simulink model "monitor"  (R2022a)
settings: Solver=FixedStepDiscrete  StartTime=0.0  StopTime=simTime  RelTol=1e-3
libraries: dspsrcs4 x16
settings Model: DataTypeOverride=Off  Creator=alpha  LastModifiedBy=alpha
settings SolverCC: AlgebraicLoopSolver=TrustRegion
settings DataIOCC: LimitDataPoints=on  SaveOutput=off  SaveTime=off
settings OptimizationCC: BlockReduction=off  ConditionallyExecuteInputs=off  DefaultParameterBehavior=Inlined  LifeSpan=inf
settings DebuggingCC: AlgebraicLoopMsg=error  SingleTaskRateTransMsg=error  UnconnectedInputMsg=warning  UnconnectedOutputMsg=warning  UnconnectedLineMsg=warning  AllowSymbolicDim=off  StrictBusMsg=ErrorOnBusTreatedAsVector  SFUnexpectedBacktrackingDiag=warning  SFNoUnconditionalDefaultTransitionDiag=warning  SFExecutionAtInitializationDiag=none  SFMachineParentedDataDiag=warning  ArithmeticOperatorsInVariantConditions=warning
settings HardwareCC: ProdBitPerPointer=32  ProdBitPerSizeT=32  ProdBitPerPtrDiffT=32  ProdLargestAtomicFloat=None  ProdIntDivRoundTo=Undefined  ProdEndianess=Unspecified  ProdWordSize=32  ProdHWDeviceType=ASIC/FPGA->ASIC/FPGA  ProdEqTarget=off
settings SFSimCC: SimUseLocalCustomCode=off  CustomCodeUndefinedFunction=UseInterfaceOnly
settings RTWCC: RTWUseLocalCustomCode=off
settings CodeAppCC: StateflowObjectComments=on
settings GRTTargetCC: TargetLangStandard=C89/C90 (ANSI)
settings ConfigComp: CovScope=ReferencedModels  CovMetricSettings=dw  CovSaveCumulativeToWorkspaceVar=on  CovSaveSingleToWorkspaceVar=on  CovExternalEMLEnable=off  CovSFcnEnable=off

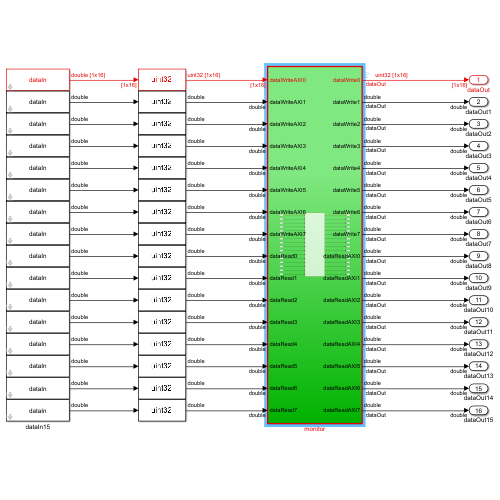
[thumbnail: Simulink's stored preview of the top-level diagram]
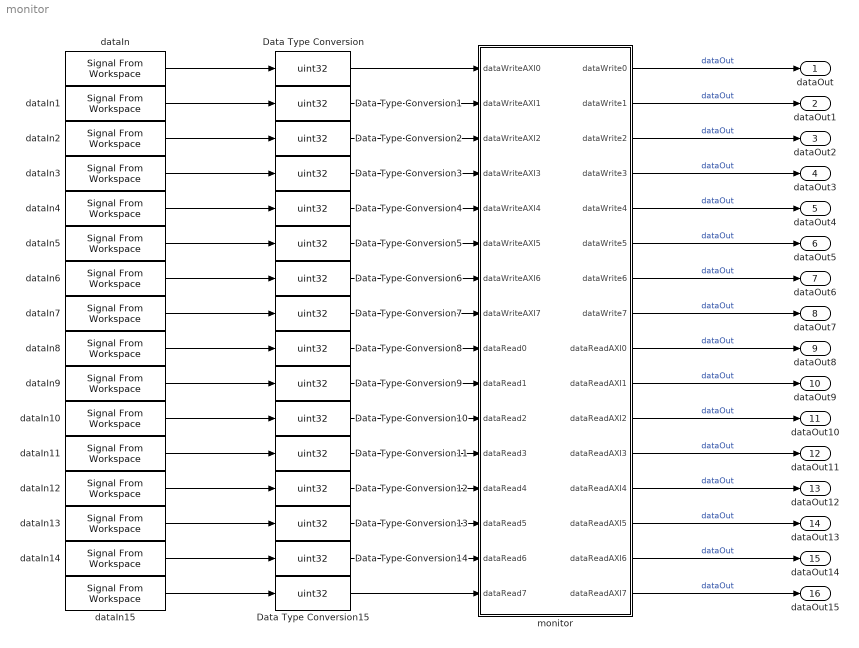
== system monitor ==
  Data Type Conversion{,1..15} (16 alike) : DataTypeConversion  OutDataTypeStr=uint32  SaturateOnIntegerOverflow=off  RndMeth=Floor
  dataIn{,1..15} (16 alike) : dspsrcs4/Signal From Workspace  X=dataIn  Ts=1  nsamps=1  OutputAfterFinalValue=Setting to zero  ignoreOrWarnInputAndFrameLengths=off  OutputFrames=off
  monitor : Subsystem  TreatAsAtomicUnit=on
  dataOut : Outport
  dataOut1 : Outport  Port=2
  dataOut2 : Outport  Port=3
  dataOut3 : Outport  Port=4
  dataOut4 : Outport  Port=5
  dataOut5 : Outport  Port=6
  dataOut6 : Outport  Port=7
  dataOut7 : Outport  Port=8
  dataOut8 : Outport  Port=9
  dataOut9 : Outport  Port=10
  dataOut10 : Outport  Port=11
  dataOut11 : Outport  Port=12
  dataOut12 : Outport  Port=13
  dataOut13 : Outport  Port=14
  dataOut14 : Outport  Port=15
  dataOut15 : Outport  Port=16
  wires:
  dataIn/1 -> Data Type Conversion/1
  Data Type Conversion/1 -> monitor/1(dataWriteAXI0)
  monitor/1(dataWrite0) -> dataOut/1  "dataOut"
  monitor/2(dataWrite1) -> dataOut1/1  "dataOut"
  monitor/3(dataWrite2) -> dataOut2/1  "dataOut"
  monitor/4(dataWrite3) -> dataOut3/1  "dataOut"
  monitor/8(dataWrite7) -> dataOut7/1  "dataOut"
  monitor/6(dataWrite5) -> dataOut5/1  "dataOut"
  monitor/5(dataWrite4) -> dataOut4/1  "dataOut"
  monitor/7(dataWrite6) -> dataOut6/1  "dataOut"
  monitor/14(dataReadAXI5) -> dataOut13/1  "dataOut"
  monitor/15(dataReadAXI6) -> dataOut14/1  "dataOut"
  monitor/12(dataReadAXI3) -> dataOut11/1  "dataOut"
  monitor/10(dataReadAXI1) -> dataOut9/1  "dataOut"
  monitor/16(dataReadAXI7) -> dataOut15/1  "dataOut"
  monitor/13(dataReadAXI4) -> dataOut12/1  "dataOut"
  monitor/9(dataReadAXI0) -> dataOut8/1  "dataOut"
  monitor/11(dataReadAXI2) -> dataOut10/1  "dataOut"
  dataIn1/1 -> Data Type Conversion1/1
  Data Type Conversion1/1 -> monitor/2(dataWriteAXI1)
  Data Type Conversion3/1 -> monitor/4(dataWriteAXI3)
  dataIn2/1 -> Data Type Conversion2/1
  Data Type Conversion2/1 -> monitor/3(dataWriteAXI2)
  dataIn3/1 -> Data Type Conversion3/1
  Data Type Conversion5/1 -> monitor/6(dataWriteAXI5)
  dataIn6/1 -> Data Type Conversion6/1
  Data Type Conversion7/1 -> monitor/8(dataWriteAXI7)
  Data Type Conversion6/1 -> monitor/7(dataWriteAXI6)
  dataIn4/1 -> Data Type Conversion4/1
  dataIn5/1 -> Data Type Conversion5/1
  dataIn7/1 -> Data Type Conversion7/1
  Data Type Conversion4/1 -> monitor/5(dataWriteAXI4)
  dataIn15/1 -> Data Type Conversion15/1
  Data Type Conversion9/1 -> monitor/10(dataRead1)
  dataIn13/1 -> Data Type Conversion13/1
  dataIn14/1 -> Data Type Conversion14/1
  Data Type Conversion13/1 -> monitor/14(dataRead5)
  Data Type Conversion12/1 -> monitor/13(dataRead4)
  Data Type Conversion15/1 -> monitor/16(dataRead7)
  Data Type Conversion14/1 -> monitor/15(dataRead6)
  dataIn10/1 -> Data Type Conversion10/1
  Data Type Conversion11/1 -> monitor/12(dataRead3)
  dataIn8/1 -> Data Type Conversion8/1
  Data Type Conversion10/1 -> monitor/11(dataRead2)
  dataIn9/1 -> Data Type Conversion9/1
  dataIn11/1 -> Data Type Conversion11/1
  dataIn12/1 -> Data Type Conversion12/1
  Data Type Conversion8/1 -> monitor/9(dataRead0)

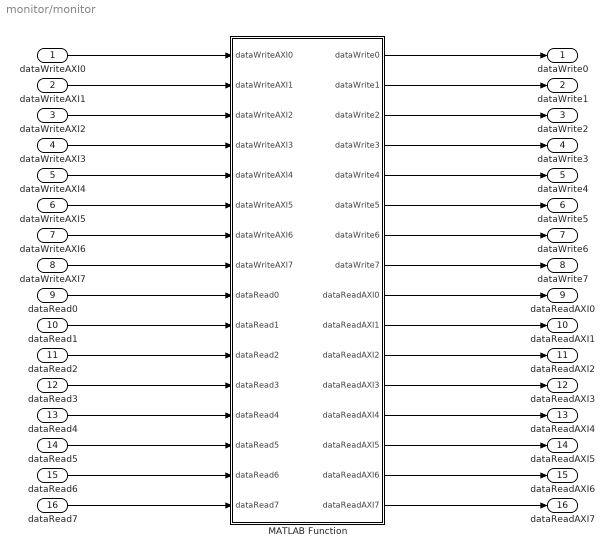
== system monitor/monitor ==
  dataWriteAXI0 : Inport
  dataWriteAXI1 : Inport  Port=2
  dataWriteAXI2 : Inport  Port=3
  dataWriteAXI3 : Inport  Port=4
  dataWriteAXI4 : Inport  Port=5
  dataWriteAXI5 : Inport  Port=6
  dataWriteAXI6 : Inport  Port=7
  dataWriteAXI7 : Inport  Port=8
  dataRead0 : Inport  Port=9
  dataRead1 : Inport  Port=10
  dataRead2 : Inport  Port=11
  dataRead3 : Inport  Port=12
  dataRead4 : Inport  Port=13
  dataRead5 : Inport  Port=14
  dataRead6 : Inport  Port=15
  dataRead7 : Inport  Port=16
  MATLAB Function : MATLAB Function  TreatAsAtomicUnit=on
  dataWrite0 : Outport
  dataWrite1 : Outport  Port=2
  dataWrite2 : Outport  Port=3
  dataWrite3 : Outport  Port=4
  dataWrite4 : Outport  Port=5
  dataWrite5 : Outport  Port=6
  dataWrite6 : Outport  Port=7
  dataWrite7 : Outport  Port=8
  dataReadAXI0 : Outport  Port=9
  dataReadAXI1 : Outport  Port=10
  dataReadAXI2 : Outport  Port=11
  dataReadAXI3 : Outport  Port=12
  dataReadAXI4 : Outport  Port=13
  dataReadAXI5 : Outport  Port=14
  dataReadAXI6 : Outport  Port=15
  dataReadAXI7 : Outport  Port=16
  wires:
  dataWriteAXI0/1 -> MATLAB Function/1(dataWriteAXI0)
  MATLAB Function/1(dataWrite0) -> dataWrite0/1
  dataWriteAXI1/1 -> MATLAB Function/2(dataWriteAXI1)
  dataWriteAXI2/1 -> MATLAB Function/3(dataWriteAXI2)
  dataWriteAXI3/1 -> MATLAB Function/4(dataWriteAXI3)
  dataWriteAXI4/1 -> MATLAB Function/5(dataWriteAXI4)
  dataWriteAXI5/1 -> MATLAB Function/6(dataWriteAXI5)
  dataWriteAXI6/1 -> MATLAB Function/7(dataWriteAXI6)
  dataWriteAXI7/1 -> MATLAB Function/8(dataWriteAXI7)
  dataRead0/1 -> MATLAB Function/9(dataRead0)
  dataRead1/1 -> MATLAB Function/10(dataRead1)
  dataRead2/1 -> MATLAB Function/11(dataRead2)
  dataRead3/1 -> MATLAB Function/12(dataRead3)
  dataRead4/1 -> MATLAB Function/13(dataRead4)
  dataRead5/1 -> MATLAB Function/14(dataRead5)
  dataRead6/1 -> MATLAB Function/15(dataRead6)
  dataRead7/1 -> MATLAB Function/16(dataRead7)
  MATLAB Function/2(dataWrite1) -> dataWrite1/1
  MATLAB Function/3(dataWrite2) -> dataWrite2/1
  MATLAB Function/4(dataWrite3) -> dataWrite3/1
  MATLAB Function/6(dataWrite5) -> dataWrite5/1
  MATLAB Function/8(dataWrite7) -> dataWrite7/1
  MATLAB Function/5(dataWrite4) -> dataWrite4/1
  MATLAB Function/7(dataWrite6) -> dataWrite6/1
  MATLAB Function/9(dataReadAXI0) -> dataReadAXI0/1
  MATLAB Function/10(dataReadAXI1) -> dataReadAXI1/1
  MATLAB Function/12(dataReadAXI3) -> dataReadAXI3/1
  MATLAB Function/11(dataReadAXI2) -> dataReadAXI2/1
  MATLAB Function/14(dataReadAXI5) -> dataReadAXI5/1
  MATLAB Function/13(dataReadAXI4) -> dataReadAXI4/1
  MATLAB Function/16(dataReadAXI7) -> dataReadAXI7/1
  MATLAB Function/15(dataReadAXI6) -> dataReadAXI6/1

== matlab function monitor/MATLAB Function ==
  data: dataWrite0 output; dataWriteAXI0 input; dataWriteAXI1 input; dataWriteAXI2 input; dataWriteAXI3 input; dataWriteAXI4 input; dataWriteAXI5 input; dataWriteAXI6 input; dataWrite1 output; dataWrite2 output; dataWrite3 output; dataWrite4 output; dataWrite5 output; dataWrite6 output; dataWrite7 output; dataWriteAXI7 input; dataRead0 input; dataRead1 input; dataRead2 input; dataRead3 input; dataRead4 input; dataRead5 input; dataRead6 input; dataRead7 input; dataReadAXI0 output; dataReadAXI1 output; dataReadAXI2 output; dataReadAXI3 output; dataReadAXI4 output; dataReadAXI5 output; dataReadAXI6 output; dataReadAXI7 output
function [dataWrite0,dataWrite1,dataWrite2,dataWrite3,dataWrite4,dataWrite5,dataWrite6,dataWrite7, ...
    dataReadAXI0,dataReadAXI1,dataReadAXI2,dataReadAXI3,dataReadAXI4,dataReadAXI5,dataReadAXI6,dataReadAXI7] ...
        = fcn( ...
    dataWriteAXI0,dataWriteAXI1,dataWriteAXI2,dataWriteAXI3,dataWriteAXI4,dataWriteAXI5,dataWriteAXI6,dataWriteAXI7,...
    dataRead0,dataRead1,dataRead2,dataRead3,dataRead4,dataRead5,dataRead6,dataRead7)

    persistent dataWrite0_reg;
    if isempty(dataWrite0_reg)
        dataWrite0_reg = uint32(0);
    end  
    persistent dataWrite1_reg;
    if isempty(dataWrite1_reg)
        dataWrite1_reg = uint32(0);
    end  
    persistent dataWrite2_reg;
    if isempty(dataWrite2_reg)
        dataWrite2_reg = uint32(0);
    end  
    persistent dataWrite3_reg;
    if isempty(dataWrite3_reg)
        dataWrite3_reg = uint32(0);
    end  
    persistent dataWrite4_reg;
    if isempty(dataWrite4_reg)
        dataWrite4_reg = uint32(0);
    end  
    persistent dataWrite5_reg;
    if isempty(dataWrite5_reg)
        dataWrite5_reg = uint32(0);
    end  
    persistent dataWrite6_reg;
    if isempty(dataWrite6_reg)
        dataWrite6_reg = uint32(0);
    end      
    persistent dataWrite7_reg;
    if isempty(dataWrite7_reg)
        dataWrite7_reg = uint32(0);
    end  

    dataWrite0 = dataWrite0_reg;
    dataWrite1 = dataWrite1_reg;
    dataWrite2 = dataWrite2_reg;    
    dataWrite3 = dataWrite3_reg;
    dataWrite4 = dataWrite4_reg;
    dataWrite5 = dataWrite5_reg;
    dataWrite6 = dataWrite6_reg;
    dataWrite7 = dataWrite7_reg;

    dataWrite0_reg = dataWriteAXI0;
    dataWrite1_reg = dataWriteAXI1;
    dataWrite2_reg = dataWriteAXI2;
    dataWrite3_reg = dataWriteAXI3;
    dataWrite4_reg = dataWriteAXI4;
    dataWrite5_reg = dataWriteAXI5;
    dataWrite6_reg = dataWriteAXI6;
    dataWrite7_reg = dataWriteAXI7;

    dataReadAXI0 = dataRead0;
    dataReadAXI1 = dataRead1;
    dataReadAXI2 = dataRead2;
    dataReadAXI3 = dataRead3;
    dataReadAXI4 = dataRead4;
    dataReadAXI5 = dataRead5;
    dataReadAXI6 = dataRead6;
    dataReadAXI7 = dataRead7;
